simulink model "ssb_am_simulink_181ME174_181ME177"  (R2020b)
settings: Solver=VariableStepAuto  StartTime=0.0  StopTime=0.05  RelTol=1e-3
undefined symbols (not defined in the file): fdesignblkfcn, gcbh
libraries: simrfV2util1 x3, dspsrcs4 x2, simrfV2elements x1
settings Model: Creator=Sayak  LastModifiedBy=Sayak

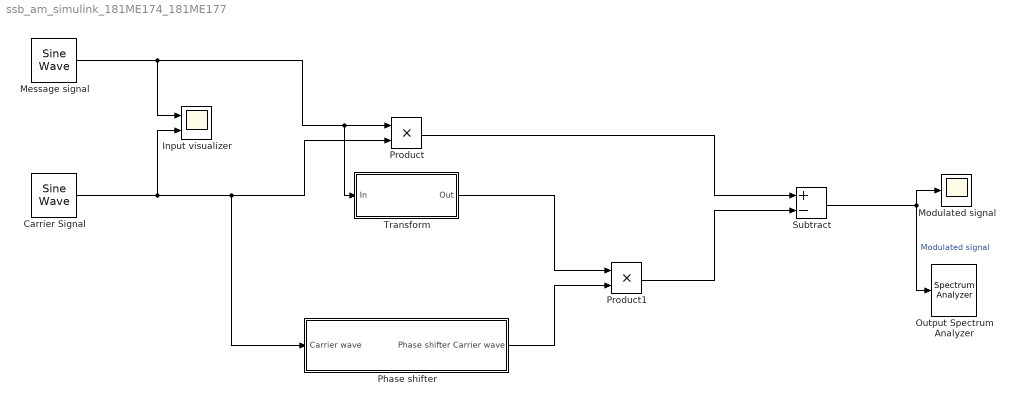
== system ssb_am_simulink_181ME174_181ME177 ==
  Carrier Signal : dspsrcs4/Sine Wave  Amplitude=1  Frequency=1000  Phase=0  SampleMode=Discrete  OutComplex=Real  CompMethod=Trigonometric fcn  TableSize=Speed  SampleTime=1/1000000  SamplesPerFrame=1  ResetState=Restart at time zero  OutputFrames=off  dataType=double  wordLen=16  udDataType=sfix(16)  fracBitsMode=Best precision  numFracBits=15  OutDataTypeStr=double  LastOutDataTypeStr=double
  Input visualizer : Scope  NumInputPorts=2
  Message signal : dspsrcs4/Sine Wave  Amplitude=1  Frequency=100  Phase=0  SampleMode=Discrete  OutComplex=Real  CompMethod=Trigonometric fcn  TableSize=Speed  SampleTime=1/1000  SamplesPerFrame=1  ResetState=Restart at time zero  OutputFrames=off  dataType=double  wordLen=16  udDataType=sfix(16)  fracBitsMode=Best precision  numFracBits=15  OutDataTypeStr=double  LastOutDataTypeStr=double
  Modulated signal : Scope
  Output Spectrum Analyzer : SpectrumAnalyzer
  Phase shifter : Subsystem
  Product : Product
  Product1 : Product
  Subtract : Sum  Inputs=+-
  Transform : Subsystem  DialogController=fdesignblkfcn  InitFcn=fdesignblkfcn(gcbh, {'InitFcn'});  mask(Hilbert Filter){}
      mask help: Design a Hilbert filter
      settings: CopyFcn=fdesignblkfcn(gcbh, {'CopyFcn'});
      mask Help: helpview(mapfilelocation('dsp'), 'dsphilbertfilter');
      mask Display: disp('Hilbert')
  wires:
  Message signal/1 -> Input visualizer/1, Product/1, Transform/1(In)
  Product/1 -> Subtract/1
  Carrier Signal/1 -> Phase shifter/1(Carrier wave), Product/2, Input visualizer/2
  Transform/1(Out) -> Product1/1
  Product1/1 -> Subtract/2
  Subtract/1 -> Modulated signal/1, Output Spectrum Analyzer/1  "Modulated signal"
  Phase shifter/1(Phase shifter Carrier wave) -> Product1/2

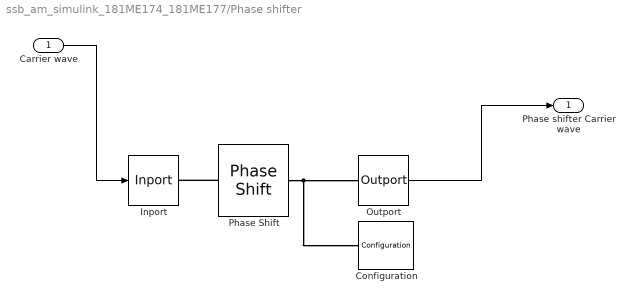
== system ssb_am_simulink_181ME174_181ME177/Phase shifter ==
  Carrier wave : Inport
  Configuration : simrfV2util1/Configuration  AutoFreq=on  Tones=[] Hz  Harmonics=[]  NormalizeCarrierPower=on  SolverType=Auto  UseCCode=on  StepSize=1e-6 s  AddNoise=on  defaultRNG=on  Seed=0  Temperature=290.0 K  SolverDelFlag=0  AbsTol=1e-6  RelTol=1e-3  MaxIter=10  ErrorEstimationType=2-norm over all variables  EnableInterpFilter=on  HiddenFIRfilterControllerParam=on  SmallSignalApprox=off  AllSimFreqs=on  SimFreqs=[] Hz  SimFreqsInternal=[]  SamplesPerFrame=1
      settings: SourceProductBaseCode=RB
  Inport : simrfV2util1/Inport  SimulinkInputSignalType=Ideal voltage  CarrierFreq=0 Hz  ZS=0  InternalGrounding=on
      settings: SourceProductBaseCode=RB
  Outport : simrfV2util1/Outport  SensorType=Ideal voltage  OutputFormat=Complex Baseband  CarrierFreq=0 Hz  ZL=Inf  InternalGrounding=on  StepSize=1e-6 s  AutoStep=on
      settings: SourceProductBaseCode=RB
  Phase Shift : simrfV2elements/Phase Shift  PhaseShift=-90 deg  InternalGrounding=on
      settings: SourceProductBaseCode=RB
  Phase shifter Carrier wave : Outport
  wires:
  Outport/1 -> Phase shifter Carrier wave/1
  Carrier wave/1 -> Inport/1
  connections:
  Phase Shift/LConn1 -- Inport/RConn1
  Phase Shift/RConn1 -- Configuration/LConn1 -- Outport/LConn1

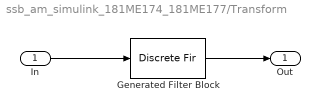
== system ssb_am_simulink_181ME174_181ME177/Transform ==
  In : Inport
  Generated Filter Block : DiscreteFir  Tag=BlockMethodSubSystem  Coefficients=[-0.026449858259791379 -0.00578355491829027 -0.016572261903348456 -0.0095390561131982743 -0.022461390535071568 -0.014999256435125952 -0.030323967074738556 -0.023012528163449009 -0.041429315821655127 -0.035762828939278346 -0.05911752381753177 -0.059034685410808696 -0.094459906652176406 -0.11739830204172252 -0.21797718993610349 -0.62869353747279177 0.62869353747279177 0.21797718993610349 0.11739830204172252 0.094459906652176406 0.059034685410808696 0.05911752381753177 0.035762828939278346 0.041429315821655127 0.023012528163449009 0.030323967074738556 0.014999256435125952 0.022461390535071568 0.0095390561131982743 0.016572261903348456 0.00578355491829027 0.026449858259791379]  InputProcessing=Columns as channels (frame based)
  Out : Outport  VectorParamsAs1DForOutWhenUnconnected=off
  wires:
  Generated Filter Block/1 -> Out/1
  In/1 -> Generated Filter Block/1
